simulink model "Flight_Simulator_v1"  (R2021a)
settings: Solver=VariableStepAuto  StartTime=0.0  StopTime=1200  RelTol=1e-3
undefined symbols (not defined in the file or in its folder): Earth, WGS84
libraries: simulink x6, aerolibconvert2 x2, aerolibfltsims x2, aerolibtransform2 x1, aerolibatmos2 x1, aerolibasang x1
settings Model: Creator=root  LastModifiedBy=Gaurav
settings SolverCC: AlgebraicLoopSolver=TrustRegion
settings DataIOCC: ReturnWorkspaceOutputs=off
settings DebuggingCC: PregeneratedLibrarySubsystemCodeDiagnostic=none  SFMachineParentedDataDiag=warning  ArithmeticOperatorsInVariantConditions=warning
settings SFSimCC: SimUseLocalCustomCode=off  CustomCodeUndefinedFunction=UseInterfaceOnly
settings RTWCC: RTWUseLocalCustomCode=off
settings CodeAppCC: StateflowObjectComments=on

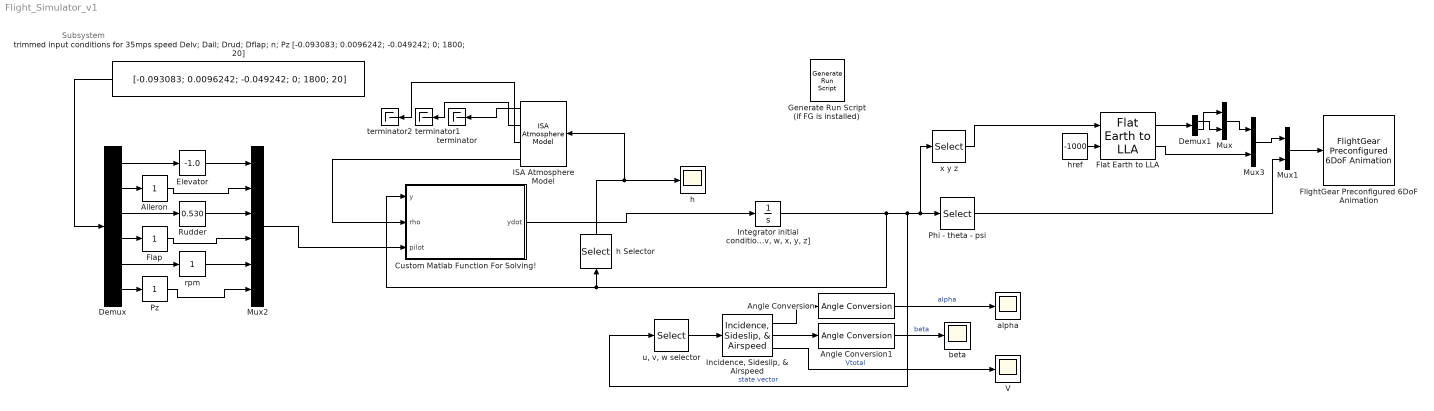
== system Flight_Simulator_v1 ==
  note: Subsystem
  Aileron : simulink/Math Operations/Slider Gain  gain=1  low=-1  high=2
  Angle Conversion : aerolibconvert2/Angle Conversion  IU=rad  OU=deg
  Angle Conversion1 : aerolibconvert2/Angle Conversion  IU=rad  OU=deg
  Custom Matlab Function For Solving! : MATLAB Function  TreatAsAtomicUnit=on
  Demux : Demux  Outputs=6
  Demux1 : Demux  Outputs=2
  Elevator : simulink/Math Operations/Slider Gain  gain=-1.0  low=-1  high=2
  Flap : simulink/Math Operations/Slider Gain  gain=1  low=-1  high=2
  Flat Earth to LLA : aerolibtransform2/Flat Earth to LLA  units=Metric (MKS)  ptype=Earth (WGS84)  F=1/298.257223563  R=6378137  refPosPort=off  LL0=[37.61 -122.39]  psi=0
  FlightGear Preconfigured 6DoF Animation : aerolibfltsims/FlightGear Preconfigured 6DoF Animation  xFlightGearVersion=v2017.3  DestinationIpAddress=127.0.0.1  DestinationPort=5502  SampleTime=1/30  packetVersion=24
  Generate Run Script (if FG is installed) : aerolibfltsims/Generate Run Script  Architecture=Win64  dataFlow=Send  GeometryModelName=dhc2F  AirportId=KSFO  RunwayId=10L  InitialAltitude=7224  InitialHeading=113  OffsetDistance=4.72  OffsetAzimuth=0  InstallScenery=off  DisableShaders=on  OriginAddress=127.0.0.1  DestinationPort=5502  OriginPort=5505  LocalAddress=127.0.0.1  OutputFileName=runfg.bat  FlightGearBaseDirectory=D:\FlightGear 2020.3
  ISA Atmosphere Model : aerolibatmos2/ISA Atmosphere Model  custom=off  g=9.80665  gamma=1.4  R=287.0531  L=0.0065  h_trop=11000  h_strat=20000  rho0=1.225  P0=101325  T0=288.15  h0=0
  "Incidence, Sideslip, & Airspeed" : aerolibasang/Incidence, Sideslip, & Airspeed
  "Integrator initial conditions for the trim state at 35mps speed [0, 0, 0, 0, 0.1919, 0, 34.2142, -0.7233, 7.3394, 0, 0,609.6] [p, q, r, phi, theta, psi, u, v, w, x, y, z]" : Integrator  InitialCondition=[0, 0, 0, 0, 0.1919, 0, 34.2142, -0.7233, 7.3394, 0, 0,609.6]
  Mux : Mux  Inputs=2
  Mux1 : Mux  Inputs=2
  Mux2 : Mux  Inputs=6
  Mux3 : Mux  Inputs=2
  Phi - theta - psi : Selector  InputPortWidth=12  IndexOptions=Index vector (dialog)  Indices=[4:6]  OutputSizes=1
  Pz : simulink/Math Operations/Slider Gain  gain=1  low=-1  high=2
  Rudder : simulink/Math Operations/Slider Gain  gain=0.530  low=-1  high=2
  V : Scope
  alpha : Scope
  beta : Scope
  h : Scope
  h Selector : Selector  InputPortWidth=12  IndexOptions=Index vector (dialog)  Indices=[12]  OutputSizes=1
  href : Constant  Value=-1000
  rpm : simulink/Math Operations/Slider Gain  gain=1  low=-1  high=2
  terminator : Terminator
  terminator1 : Terminator
  terminator2 : Terminator
  trimmed input conditions for 35mps speed Delv; Dail; Drud; Dflap; n; Pz [-0.093083; 0.0096242; -0.049242; 0; 1800; 20] : Constant  Value=[-0.093083; 0.0096242; -0.049242; 0; 1800; 20]
  "u, v, w selector" : Selector  InputPortWidth=12  IndexOptions=Index vector (dialog)  Indices=[7,8,9]  OutputSizes=1
  x y z : Selector  InputPortWidth=12  IndexOptions=Index vector (dialog)  Indices=[10,11,12]  OutputSizes=1
  wires:
  "Integrator initial conditions for the trim state at 35mps speed [0, 0, 0, 0, 0.1919, 0, 34.2142, -0.7233, 7.3394, 0, 0,609.6] [p, q, r, phi, theta, psi, u, v, w, x, y, z]"/1 -> Phi - theta - psi/1, x y z/1, "u, v, w selector"/1, h Selector/1, Custom Matlab Function For Solving!/1(y)  "state vector"
  Custom Matlab Function For Solving!/1(ydot) -> "Integrator initial conditions for the trim state at 35mps speed [0, 0, 0, 0, 0.1919, 0, 34.2142, -0.7233, 7.3394, 0, 0,609.6] [p, q, r, phi, theta, psi, u, v, w, x, y, z]"/1
  Phi - theta - psi/1 -> Mux1/2
  "u, v, w selector"/1 -> "Incidence, Sideslip, & Airspeed"/1
  "Incidence, Sideslip, & Airspeed"/1 -> Angle Conversion/1
  "Incidence, Sideslip, & Airspeed"/3 -> V/1  "Vtotal"
  Angle Conversion/1 -> alpha/1  "alpha"
  trimmed input conditions for 35mps speed Delv; Dail; Drud; Dflap; n; Pz [-0.093083; 0.0096242; -0.049242; 0; 1800; 20]/1 -> Demux/1
  h Selector/1 -> ISA Atmosphere Model/1, h/1
  ISA Atmosphere Model/4 -> Custom Matlab Function For Solving!/2(rho)
  ISA Atmosphere Model/3 -> terminator2/1
  ISA Atmosphere Model/2 -> terminator1/1
  ISA Atmosphere Model/1 -> terminator/1
  Angle Conversion1/1 -> beta/1  "beta"
  "Incidence, Sideslip, & Airspeed"/2 -> Angle Conversion1/1
  x y z/1 -> Flat Earth to LLA/1
  href/1 -> Flat Earth to LLA/2
  Mux1/1 -> FlightGear Preconfigured 6DoF Animation/1
  Mux2/1 -> Custom Matlab Function For Solving!/3(pilot)
  Demux/1 -> Elevator/1
  Demux/2 -> Aileron/1
  Demux/3 -> Rudder/1
  Demux/4 -> Flap/1
  Demux/5 -> rpm/1
  Demux/6 -> Pz/1
  Elevator/1 -> Mux2/1
  Aileron/1 -> Mux2/2
  Rudder/1 -> Mux2/3
  Flap/1 -> Mux2/4
  rpm/1 -> Mux2/5
  Pz/1 -> Mux2/6
  Flat Earth to LLA/2 -> Mux3/2
  Demux1/1 -> Mux/2
  Mux/1 -> Mux3/1
  Demux1/2 -> Mux/1
  Mux3/1 -> Mux1/1
  Flat Earth to LLA/1 -> Demux1/1

== matlab function Flight_Simulator_v1/Custom Matlab Function For Solving! ==
  data: ydot output; y input; rho input; pilot input
function ydot = fcn(y, rho, pilot)
%odefun calculates the time rates to be used in ode45 function
%   Detailed explanation goes here
% y = [p,q,r,phi,theta,psi,u,v,w,x,y,z]

    Ix = 5368.39; Iy = 6.92893e3; Iz = 11158.75;
    Ixy = 0; Ixz = 1.1764e2; Iyz = 0;
    m = 2288.231; g = 9.81;
    
    %%
    data = load('dhc2_vars.mat');
    
    %%
    %inputs and input vector U
    
    Delv = pilot(1); Dail = pilot(2); Drud = pilot(3); Dflap = pilot(4);
    n = pilot(5); Pz = pilot(6);
    
    %%
    % y = [p,q,r,phi,theta,psi,u,v,w,x,y,z]
    %      1,2,3,4,   5   ,6  ,7,8,9,10,11,12
    p = y(1); q = y(2); r = y(3); phi = y(4); theta = y(5); psi = y(6);
    u = y(7); v = y(8); w = y(9); z = y(12);
    V = sqrt(u^2 + v^2 + w^2);
    alpha = atan2(w,u);
    beta = asin(v/V);
    
    P = 0.7355*(-326.5+(0.00412*(Pz+7.4)*(n+2010)+(408-0.0965*n)*(1-rho/1.225)));
    dpt=0.08696+191.18*(P*2/rho/V^3);
    qdyn=0.5*rho*V^2;
    
    Cx = data.Cx0+data.Cx_alpha*alpha+data.Cx_alpha2*alpha^2+data.Cx_alpha3*alpha^3+data.Cx_q*q*data.beaver_c/V...
         + data.Cx_dr*Drud+data.Cx_df*Dflap+data.Cx_df_alpha*alpha*Dflap...
         + data.Cx_dpt*dpt+data.Cx_dpt2_alpha*dpt^2*alpha;

    Cy = data.Cy0+data.Cy_beta*beta+data.Cy_p*p*data.beaver_b/2/V+data.Cy_r*r*data.beaver_b/2/V...
         + data.Cy_da*Dail+data.Cy_dr*Drud+data.Cy_dr_alpha*alpha*Drud;

    Cz = data.Cz0+data.Cz_alpha*alpha+data.Cz_alpha3*alpha^3+data.Cz_q*q*data.beaver_c/V+data.Cz_de*Delv...
         + data.Cz_de_beta*Delv*beta^2+data.Cz_df*Dflap...
         + data.Cz_df_alpha*alpha*Dflap+data.Cz_dpt*dpt;

    Cl = data.Cl0+data.Cl_beta*beta+data.Cl_p*p*data.beaver_b/2/V+data.Cl_r*r*data.beaver_b/2/V...
         + data.Cl_da*Dail+data.Cl_dr*Drud...
         + data.Cl_da_alpha*alpha*Dail+data.Cl_alpha2_dpt*alpha^2*dpt;

    Cm = data.Cm0+data.Cm_alpha*alpha+data.Cm_alpha2*alpha^2+data.Cm_q*q*data.beaver_c/V...
         + data.Cm_de*Delv+data.Cm_beta2*beta^2+data.Cm_r*r*data.beaver_b/2/V+data.Cm_df*Dflap...
         + data.Cm_dpt*dpt;

    Cn = data.Cn0+data.Cn_beta*beta+data.Cn_p*p*data.beaver_b/2/V+data.Cn_r*r*data.beaver_b/2/V+data.Cn_da...
         *Dail+data.Cn_dr*Drud+data.Cn_q*q*data.beaver_c/V+data.Cn_beta3*beta^3+data.Cn_dpt3*dpt^3;

    Fx = Cx*qdyn*data.beaver_S;
    Fy = Cy*qdyn*data.beaver_S;
    Fz = Cz*qdyn*data.beaver_S;
    L = Cl*qdyn*data.beaver_S*data.beaver_b;
    M = Cm*qdyn*data.beaver_S*data.beaver_c;
    N = Cn*qdyn*data.beaver_S*data.beaver_b;

        
    %%
    ydot = nan(12,1);
    
    % Hisham Method [Wrong]
%     ydot(1) = (Iz*L + Ixz*N + Ixz^2*q*r - Iz^2*q*r - Ixz*Iy*p*q + 2*Ixz*Iz*p*q + Iy*Iz*q*r)/(Ixz^2 + Ix*Iz);
%     
%     ydot(2) = (M - Ixz*p^2 + Ixz*r^2 - Ix*q*r + Iz*q*r)/Iy;
%     
%     ydot(3) = -(Ixz*L - Ix*N + Ixz^2*p*q + Ix*Iy*p*q - Ix*Iz*p*q - Ix*Ixz*q*r + Ixz*Iy*q*r - Ixz*Iz*q*r)/(Ixz^2 + Ix*Iz);
    
    % Khaled Method
    ydot(1) = (Iz*L + Ixz*N - Ixz^2*q*r - Iz^2*q*r - Ixz*Iy*p*q +Ixz*Iz*p*q+Ixz*Ix*p*q+ Iy*Iz*q*r)/(Ix*Iz-Ixz^2);
    
    ydot(2) = (M - Ixz*p^2 + Ixz*r^2 - Ix*p*r + Iz*p*r)/Iy;
    
    ydot(3) = (Ixz*L + Ix*N + Ix^2*p*q - Ix*Iy*p*q - Ixz^2*p*q - Ix*Ixz*q*r + Ixz*Iy*q*r - Ixz*Iz*q*r)/(Ix*Iz-Ixz^2);
    
    %%
    euler = [[1, sin(y(4))*tan(y(5)), cos(y(4))*tan(y(5))];...
             [0, cos(y(4)), -sin(y(4))];...
             [0, sin(y(4))*(1/cos(y(5))), cos(y(4))*(1/cos(y(5)))]] * ...
             [y(1); y(2); y(3)];
    
    ydot(4) = euler(1);
    ydot(5) = euler(2);
    ydot(6) = euler(3);

%     ydot(4) = p + r*cos(phi)*tan(theta) + q*sin(phi)*tan(theta);
%     ydot(5) = q*cos(phi) - r*sin(phi);
%     ydot(6) = (r*cos(phi))/cos(theta) + (q*sin(phi))/cos(theta);
    
    %%
    ydot(7) = (Fx - g*m*sin(theta) - m*q*w + m*r*v)/m;
    ydot(8) = (Fy + m*p*w - m*r*u + g*m*cos(theta)*sin(phi))/m;
    ydot(9) = (Fz - m*p*v + m*q*u + g*m*cos(phi)*cos(theta))/m;
    
    %%
    C = [[cos(y(5))*cos(y(6)), sin(y(4))*sin(y(5))*cos(y(6))-(cos(y(4))*sin(y(6))), cos(y(4))*sin(y(5))*cos(y(6))+(sin(y(4))*sin(y(6)))];
         [cos(y(5))*sin(y(6)), sin(y(4))*sin(y(5))*sin(y(6))+(cos(y(4))*cos(y(6))), cos(y(4))*sin(y(5))*sin(y(6))-(sin(y(4))*cos(y(6)))];
         [-sin(y(5)), sin(y(4))*cos(y(5)), cos(y(4))*cos(y(5))]];
    
    Cmat = C * [y(7); y(8); y(9)];
    
    ydot(10) = Cmat(1);
    ydot(11) = Cmat(2);
    ydot(12) = Cmat(3);
    
%     ydot(10) = w*(sin(phi)*sin(psi) + cos(psi)^2*sin(theta)) - v*(cos(phi)*sin(psi) - cos(psi)*sin(phi)*sin(theta)) + u*cos(psi)*cos(theta);
%     ydot(11) = v*(cos(phi)*cos(psi) + sin(phi)*sin(psi)*sin(theta)) - w*(cos(psi)*sin(phi) - cos(phi)*sin(psi)*sin(theta)) + u*cos(theta)*sin(psi);
%     ydot(12) = w*cos(phi)*cos(theta) - u*sin(theta) + v*cos(theta)*sin(phi);

    ydot = [ydot(1); ydot(2); ydot(3); ydot(4); ydot(5); ydot(6);...
            ydot(7); ydot(8); ydot(9); ydot(10); ydot(11); ydot(12)];
end
